simulink model "satellite_sim"  (R2016b)
settings: Solver=ode45  StartTime=0.0  StopTime=200  RelTol=1e-3  EnableMultiTasking=on
InitFcn:
  | addpath ./..
  | satelliteParam
  | satelliteParamHW10
undefined symbols (not defined in the file or in its folder): P, satellite_animation, satellite_ctrl
settings Model: Creator=beard  LastModifiedBy=beard
settings DataIOCC: LimitDataPoints=on  SaveFormat=Array  SignalLoggingSaveFormat=ModelDataLogs
settings OptimizationCC: ExpressionDepthLimit=2147483647  InitFltsAndDblsToZero=on  LifeSpan=inf
settings DebuggingCC: UnderspecifiedInitializationDetection=Classic  MergeDetectMultiDrivingBlocksExec=none  SolverPrmCheckMsg=warning  FcnCallInpInsideContextMsg=warning  StateNameClashWarn=warning  SFUnexpectedBacktrackingDiag=warning  SFNoUnconditionalDefaultTransitionDiag=warning  SFExecutionAtInitializationDiag=none
settings HardwareCC: ProdBitPerPointer=32  ProdBitPerSizeT=32  ProdBitPerPtrDiffT=32  ProdLargestAtomicFloat=None  ProdIntDivRoundTo=Undefined  ProdEndianess=Unspecified  ProdWordSize=32  ProdHWDeviceType=32-bit Generic
settings ModelReferenceCC: PropagateSignalLabelsOutOfModel=off
settings GRTTargetCC: TargetLangStandard=C89/C90 (ANSI)  GeneratePreprocessorConditionals=Disable all  CombineOutputUpdateFcns=off  GRTInterface=on
settings ConfigComp: CovMetricSettings=dw  CovHtmlReporting=on  CovSaveCumulativeToWorkspaceVar=on  CovSaveSingleToWorkspaceVar=on  CovExternalEMLEnable=off

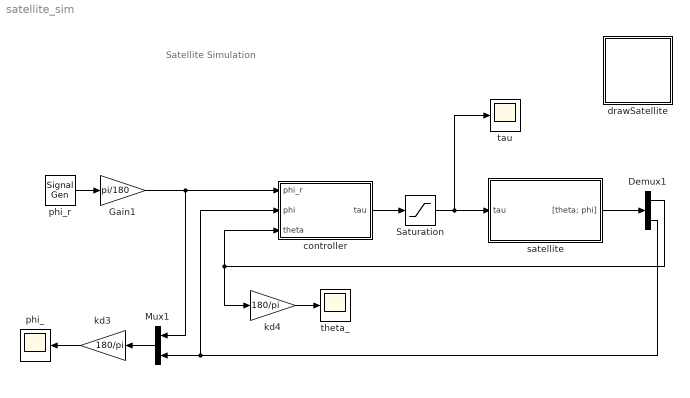
== system satellite_sim ==
  note: Satellite Simulation
  Demux1 : Demux  Outputs=2
  Gain1 : Gain  Gain=pi/180
  Mux1 : Mux  Inputs=2
  Saturation : Saturate  UpperLimit=P.taumax  LowerLimit=-P.taumax
  controller : Subsystem
  drawSatellite : Subsystem
      mask Display: image(imread('tv.jpg'))
  kd3 : Gain  Gain=180/pi
  kd4 : Gain  Gain=180/pi
  phi_ : Scope
  phi_r : SignalGenerator  WaveForm=square  Amplitude=15  Frequency=.015
  satellite : Subsystem
  tau : Scope
  theta_ : Scope
  wires:
  satellite/1("[theta; phi]") -> Demux1/1
  phi_r/1 -> Gain1/1
  Saturation/1 -> satellite/1(tau), tau/1
  Demux1/1 -> controller/3(theta), kd4/1
  controller/1(tau) -> Saturation/1
  Mux1/1 -> kd3/1
  kd3/1 -> phi_/1
  Demux1/2 -> controller/2(phi), Mux1/2
  Gain1/1 -> Mux1/1, controller/1(phi_r)
  kd4/1 -> theta_/1

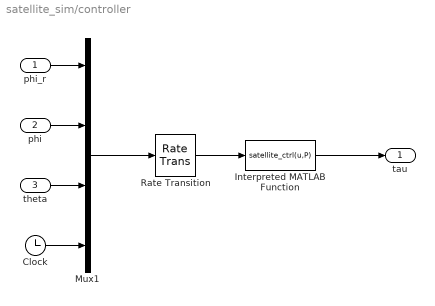
== system satellite_sim/controller ==
  phi_r : Inport
  phi : Inport  Port=2
  theta : Inport  Port=3
  Clock : Clock
  Interpreted MATLAB Function : MATLABFcn  MATLABFcn=satellite_ctrl(u,P)  OutputDimensions=1
  Mux1 : Mux
  Rate Transition : RateTransition  OutPortSampleTime=P.Ts
  tau : Outport
  wires:
  Mux1/1 -> Rate Transition/1
  phi_r/1 -> Mux1/1
  Interpreted MATLAB Function/1 -> tau/1
  Clock/1 -> Mux1/4
  Rate Transition/1 -> Interpreted MATLAB Function/1
  theta/1 -> Mux1/3
  phi/1 -> Mux1/2

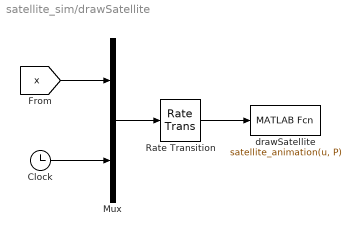
== system satellite_sim/drawSatellite ==
  Clock : Clock
  Mux : Mux  Inputs=2
  Rate Transition : RateTransition  OutPortSampleTime=P.t_plot
  drawSatellite : MATLABFcn  MATLABFcn=satellite_animation(u, P)  OutputDimensions=0
  wires:
  Rate Transition/1 -> drawSatellite/1
  Clock/1 -> Mux/2
  [x] -> Mux/1
  Mux/1 -> Rate Transition/1

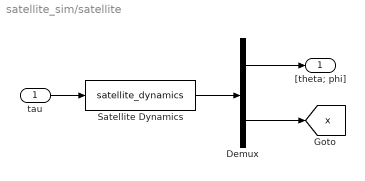
== system satellite_sim/satellite ==
  tau : Inport
  Demux : Demux  Outputs=[2;4]
  Satellite Dynamics : S-Function  FunctionName=satellite_dynamics  Parameters=P  SFunctionDeploymentMode=off  EnableBusSupport=off
  "[theta; phi]" : Outport
  tag scope: x=global
  wires:
  tau/1 -> Satellite Dynamics/1
  Satellite Dynamics/1 -> Demux/1
  Demux/1 -> "[theta; phi]"/1
  Demux/2 -> [x]
